simulink model "Project2_Week2_Simulink"  (R2023b)
settings: Solver=VariableStepAuto  StartTime=0.0  StopTime=10.0  RelTol=1e-3
settings Model: Creator=Conor  LastModifiedBy=Conor

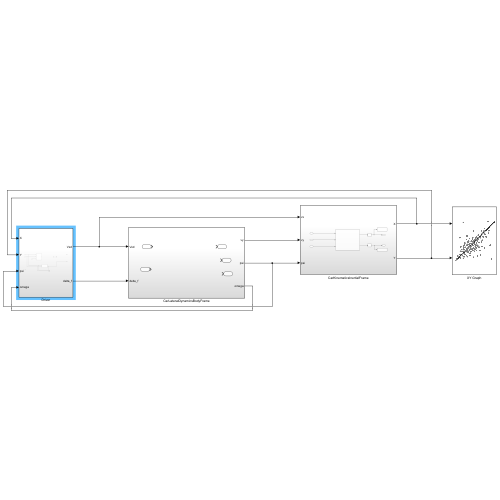
[thumbnail: Simulink's stored preview of the top-level diagram]
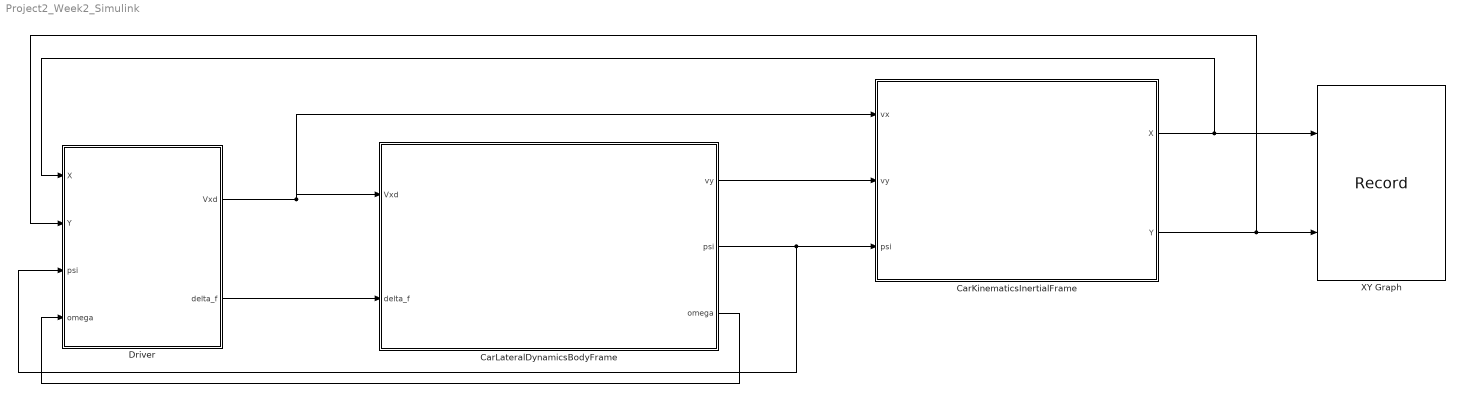
== system Project2_Week2_Simulink ==
  CarKinematicsInertialFrame : Subsystem
  CarLateralDynamicsBodyFrame : Subsystem
  Driver : Subsystem
  XY Graph : Record  FileSettingsInternal="{\"entries\":[{\"content\":{\"excelSettings\":{\"content\":{},\"type\":\"Streamout.ExcelSettings\"}},\"type\":\"Streamout.FileSettingStorage\",\"uuid\":\"\"}],\"packageUris\":[\"http:\\/\\/schema.mathworks.com\\/mf0\\/streamout_blocks\\/R2020a\"],\"version\":\"1.0\"}"  Layout=[1 1]  SignalsInternal="{\"entries\":[{\"content\":{\"signals\":[{\"content\":{\"blockPath\":[],\"dimensions\":[1],\"domain\":\"\",\"lineColor\":\"#a2142f\",\"plots\":[1],\"port\":1,\"signalID\":16,\"signalName\":\"XY Graph:1\"},\"type\":\"RecordBlkView.Signal\",\"uuid\":\"\"},{\"content\":{\"blockPath\":[],\"dimensions\":[1],\"domain\":\"\",\"lineColor\":\"#139fff\",\"plots\":[1],\"port\":2,\"signalID\":19,\"signalName\":\"XY Graph:2\"},\"type\":\"RecordBlkView.Signal\",\"uuid\":\"\"}]},\"type\":\"RecordBlkView.InputSignals\",\"uuid\":\"\"}],\"packageUris\":[\"http:\\/\\/schema.mathworks.com\\/mf0\\/streamout_blocks\\/R2020a\"],\"version\":\"1.0\"}"  VisualizationBindings="{\"xyplotplugin\":{\"info\":[{\"series\":[{\"bindingParametersList\":[{\"parameter\":\"X-Axis\",\"signalID\":16,\"signalName\":\"XY Graph:1\"},{\"parameter\":\"Y-Axis\",\"signalID\":19,\"signalName\":\"XY Graph:2\"}],\"seriesID\":10423}],\"subplotID\":1}]}}"  CompatibilityTag=XY
  wires:
  CarKinematicsInertialFrame/1(X) -> Driver/1(X), XY Graph/1
  CarKinematicsInertialFrame/2(Y) -> Driver/2(Y), XY Graph/2
  Driver/2(delta_f) -> CarLateralDynamicsBodyFrame/2(delta_f)
  Driver/1(Vxd) -> CarKinematicsInertialFrame/1(vx), CarLateralDynamicsBodyFrame/1(Vxd)
  CarLateralDynamicsBodyFrame/2(psi) -> Driver/3(psi), CarKinematicsInertialFrame/3(psi)
  CarLateralDynamicsBodyFrame/1(vy) -> CarKinematicsInertialFrame/2(vy)
  CarLateralDynamicsBodyFrame/3(omega) -> Driver/4(omega)

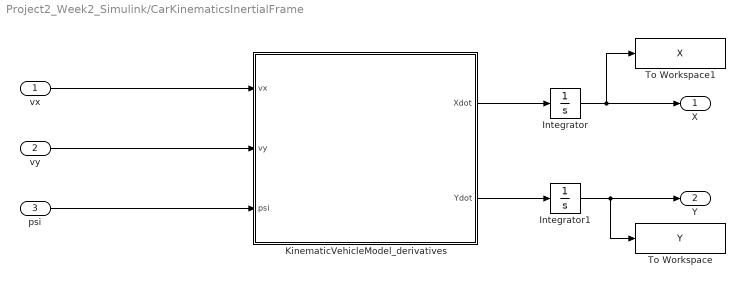
== system Project2_Week2_Simulink/CarKinematicsInertialFrame ==
  vx : Inport
  vy : Inport  Port=2
  psi : Inport  Port=3
  Integrator : Integrator
  Integrator1 : Integrator
  KinematicVehicleModel_derivatives : MATLAB Function  TreatAsAtomicUnit=on
  To Workspace : ToWorkspace  VariableName=Y  SaveFormat=Timeseries  SampleTime=-1
  To Workspace1 : ToWorkspace  VariableName=X  SaveFormat=Timeseries  SampleTime=-1
  X : Outport
  Y : Outport  Port=2
  wires:
  psi/1 -> KinematicVehicleModel_derivatives/3(psi)
  vy/1 -> KinematicVehicleModel_derivatives/2(vy)
  vx/1 -> KinematicVehicleModel_derivatives/1(vx)
  KinematicVehicleModel_derivatives/2(Ydot) -> Integrator1/1
  KinematicVehicleModel_derivatives/1(Xdot) -> Integrator/1
  Integrator1/1 -> Y/1, To Workspace/1
  Integrator/1 -> To Workspace1/1, X/1

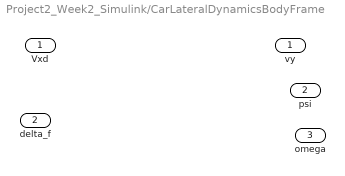
== system Project2_Week2_Simulink/CarLateralDynamicsBodyFrame ==
  Vxd : Inport
  delta_f : Inport  Port=2
  vy : Outport
  psi : Outport  Port=2
  omega : Outport  Port=3

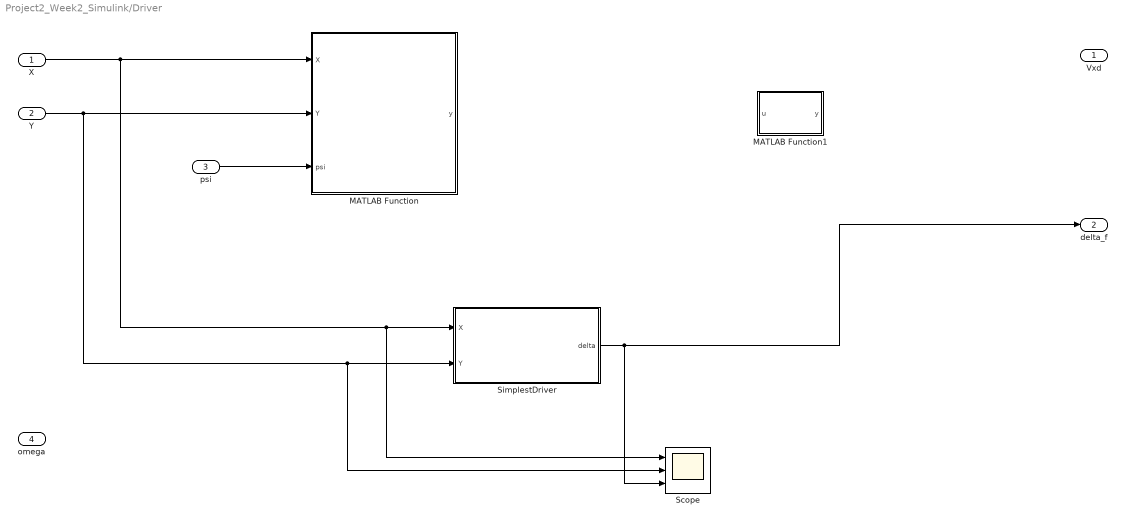
== system Project2_Week2_Simulink/Driver ==
  X : Inport
  Y : Inport  Port=2
  psi : Inport  Port=3
  omega : Inport  Port=4
  MATLAB Function : MATLAB Function  TreatAsAtomicUnit=on
  MATLAB Function1 : MATLAB Function  TreatAsAtomicUnit=on
  Scope : Scope  NumInputPorts=3
  SimplestDriver : MATLAB Function  TreatAsAtomicUnit=on
  Vxd : Outport
  delta_f : Outport  Port=2
  wires:
  Y/1 -> Scope/2, SimplestDriver/2(Y), MATLAB Function/2(Y)
  X/1 -> Scope/1, SimplestDriver/1(X), MATLAB Function/1(X)
  psi/1 -> MATLAB Function/3(psi)
  SimplestDriver/1(delta) -> Scope/3, delta_f/1

== matlab function Project2_Week2_Simulink/Driver/SimplestDriver ==
  data: X input; delta output; Y input
function delta = SimplestDriver(X, Y)

if abs(Y) < 0.5
    delta = 0;
elseif abs(Y -400) < 0.5
    delta = 0;
elseif X > 900
    delta = 5;
else
    delta = -5;
end

== matlab function Project2_Week2_Simulink/CarKinematicsInertialFrame/KinematicVehicleModel_derivatives ==
  data: vx input; Xdot output; vy input; psi input; Ydot output
function [Xdot, Ydot] = fcn(vx, vy, psi)
    temp = TF(psi) * [vx;vy];
    Xdot = temp(1);
    Ydot = temp(2);
end

function y = TF(psi)
    y = [cos(psi), - sin(psi); sin(psi), cos(psi)];
    
end

== matlab function Project2_Week2_Simulink/Driver/MATLAB Function ==
  data: X input; y output; Y input; psi input
function y = fcn(X, Y, psi)

y = u;

== matlab function Project2_Week2_Simulink/Driver/MATLAB Function1 ==
  data: u input; y output
function y = fcn(u)

y = u;
